simulink model "zad8"  (R2023a)
settings: Solver=VariableStepAuto  StartTime=0.0  StopTime=100  RelTol=1e-3
model workspace (MAT data in the model file):
  T1 = Simulink.Parameter
  T1.Value = 8
  T1.DataType = 'auto'
  T1.Complexity = 'real'
  T1.Dimensions = [1 1]
  T2 = Simulink.Parameter
  T2.Value = 9
  T2.DataType = 'auto'
  T2.Complexity = 'real'
  T2.Dimensions = [1 1]
values from neighbouring files (symbols this model uses):
  a1 = -0.8    [zad10.m]    (also in zad2.m; zad3.m)
  a2 = -0.86    [zad10.m]    (also in zad2.m; zad3.m)
  a3 = -0.41    [zad10.m]    (also in zad2.m; zad3.m)
  a4 = -0.41    [zad10.m]    (also in zad2.m; zad3.m)
  K = 1    [zad10.m]    (also in zad2.m; zad3.m)
  T1 = 9    [zad10.m]
  T2 = 8    [zad10.m]
  u_point = 0.5    [zad10.m]    (also in zad3.m = 0)
undefined symbols (not defined in the file or in its folder): DiscIntNeverNeededParam
settings Model: Creator=pkutyl  LastModifiedBy=pkutyl

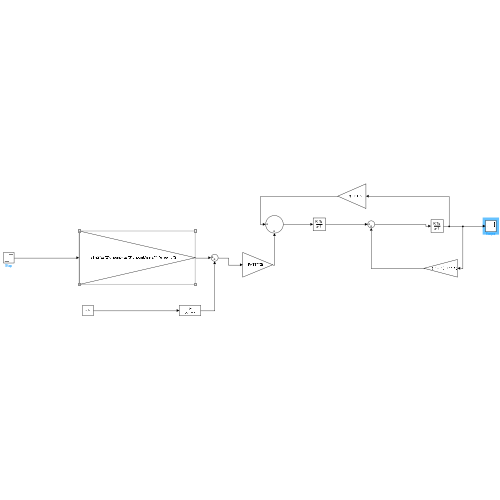
[thumbnail: Simulink's stored preview of the top-level diagram]
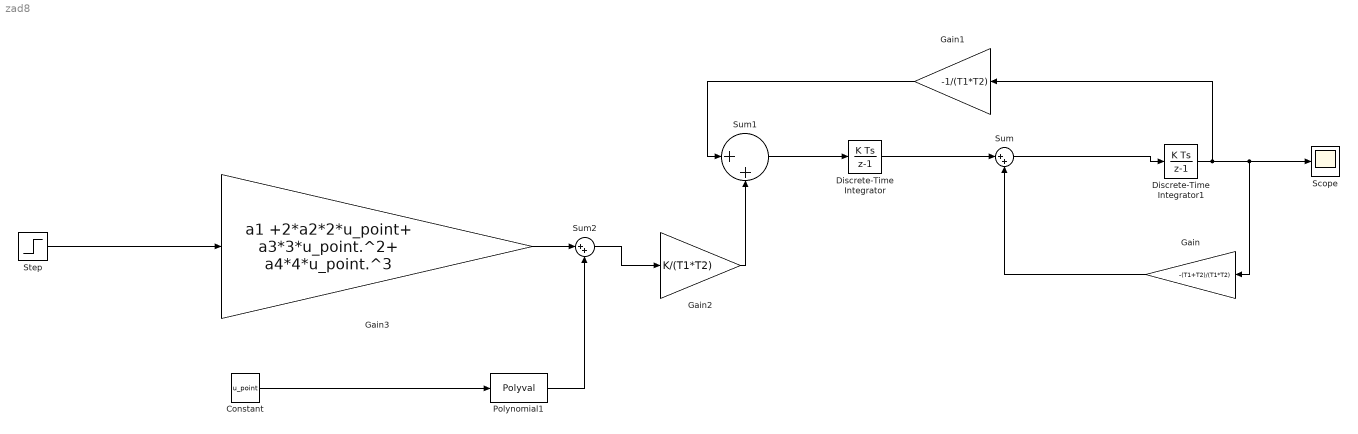
== system zad8 ==
  Constant : Constant  Value=u_point
  Discrete-Time Integrator : DiscreteIntegrator  SampleTime=-1  ICPrevOutput=DiscIntNeverNeededParam  ICPrevScaledInput=DiscIntNeverNeededParam
  Discrete-Time Integrator1 : DiscreteIntegrator  SampleTime=-1  ICPrevOutput=DiscIntNeverNeededParam  ICPrevScaledInput=DiscIntNeverNeededParam
  Gain : Gain  Gain=-(T1+T2)/(T1*T2)
  Gain1 : Gain  Gain=-1/(T1*T2)
  Gain2 : Gain  Gain=K/(T1*T2)
  Gain3 : Gain  Gain=a1 +2*a2*2*u_point+ a3*3*u_point.^2+ a4*4*u_point.^3
  Polynomial1 : Polyval  Coefs=[-3*a4, -2*a3, - a2,0,0]
  Scope : Scope
  Step : Step  SampleTime=0
  Sum : Sum  Inputs=|++
  Sum1 : Sum  Inputs=|++
  Sum2 : Sum  Inputs=|++
  wires:
  Discrete-Time Integrator/1 -> Sum/1
  Discrete-Time Integrator1/1 -> Gain1/1, Scope/1, Gain/1
  Gain1/1 -> Sum1/1
  Sum/1 -> Discrete-Time Integrator1/1
  Gain/1 -> Sum/2
  Sum1/1 -> Discrete-Time Integrator/1
  Gain2/1 -> Sum1/2
  Constant/1 -> Polynomial1/1
  Polynomial1/1 -> Sum2/2
  Sum2/1 -> Gain2/1
  Step/1 -> Gain3/1
  Gain3/1 -> Sum2/1
